simulink model "embedded_transpose"  (Simulink 7.4)
settings: Solver=ode3  StartTime=0.0  StopTime=10.0  FixedStep=1  RelTol=1e-3
settings Model: Creator=Harmon S. Nine  LastModifiedBy=Harmon S. Nine

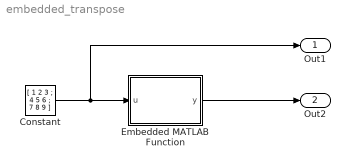
== system embedded_transpose ==
  Constant : Constant  Value=[ 1 2 3 ; 4 5 6 ; 7 8 9 ]  VectorParams1D=off  OutDataType=fixdt(1, 16)  OutScaling=2^0
  Embedded MATLAB Function : Stateflow chart
  Out1 : Outport  OutDataType=fixdt(1, 16)  OutScaling=2^0
  Out2 : Outport  Port=2  OutDataType=fixdt(1, 16)  OutScaling=2^0
  wires:
  Constant/1 -> Embedded MATLAB Function/1(u), Out1/1
  Embedded MATLAB Function/1(y) -> Out2/1

== matlab function Embedded MATLAB Function ==
  data: u input double; y output double
function y = fcn(u)
%#eml

y = transpose( u );
